simulink model "DiscreteSimulationTest"  (R2013b)
settings: Solver=ode45  StartTime=0.0  StopTime=10.0  RelTol=1e-3
libraries: simulink x2
settings Model: Creator=gyurse  LastModifiedBy=gyurse

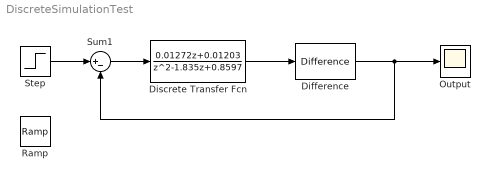
== system DiscreteSimulationTest ==
  Difference : simulink/Discrete/Difference  ICPrevInput=0.0  InputProcessing=Inherited  OutMin=[]  OutMax=[]  OutDataType=fixdt(1, 16)  OutScaling=2^-10  DoSatur=off
  Discrete Transfer Fcn : DiscreteTransferFcn  Numerator=[0.01272 0.01203]  Denominator=[1 -1.835 0.8597]  SampleTime=0.025
  Output : Scope
      settings: TimeRange=10  YMin=0  YMax=1.4
  Ramp : simulink/Sources/Ramp  slope=1  start=0  X0=0
  Step : Step  SampleTime=0
  Sum1 : Sum  Inputs=|+-
  wires:
  Step/1 -> Sum1/1
  Difference/1 -> Output/1, Sum1/2
  Sum1/1 -> Discrete Transfer Fcn/1
  Discrete Transfer Fcn/1 -> Difference/1
